simulink model "EdLuTSimulink"  (Simulink 8.1)
settings: Solver=ode3  StartTime=0.0  StopTime=1.  FixedStep=0.002  RelTol=1e-3
undefined symbols (not defined in the file or in its folder): frne
undefined symbols (not defined in the file): context, RRedKuKa, RRedKuKadet
libraries: simulink x1
(part 2 of 2)

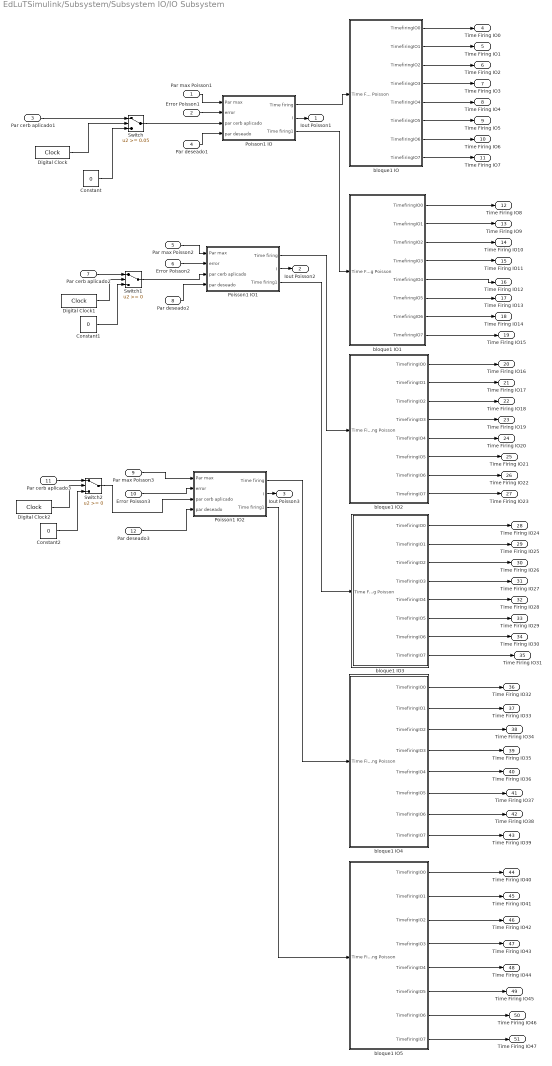
== system EdLuTSimulink/Subsystem/Subsystem IO/IO Subsystem  ==
  Par max Poisson1 : Inport
  Error Poisson1 : Inport  Port=2
  Par cerb aplicado1 : Inport  Port=3
  Par deseado1 : Inport  Port=4
  Par max Poisson2 : Inport  Port=5
  Error Poisson2 : Inport  Port=6
  Par cerb aplicado2 : Inport  Port=7
  Par deseado2 : Inport  Port=8
  Par max Poisson3 : Inport  Port=9
  Error Poisson3 : Inport  Port=10
  Par cerb aplicado3 : Inport  Port=11
  Par deseado3 : Inport  Port=12
  Constant : Constant  Value=0
  Constant1 : Constant  Value=0
  Constant2 : Constant  Value=0
  Digital Clock : DigitalClock  SampleTime=0.002
  Digital Clock1 : DigitalClock  SampleTime=0.002
  Digital Clock2 : DigitalClock  SampleTime=0.002
  Poisson1 IO : Subsystem  mask{a=0.001, b=1, timestep=0.002, firingrate=50}
      mask prompts: a "Valor a del intervalo [a b] para la generación de la poisson"; b "Valor b del intervalo [a b] para la generación de la poisson"; timestep "Tiempo de paso"
  Poisson1 IO1 : Subsystem  mask{a=0.001, b=1, timestep=0.002, firingrate=50}
      mask prompts: a "Valor a del intervalo [a b] para la generación de la poisson"; b "Valor b del intervalo [a b] para la generación de la poisson"; timestep "Tiempo de paso"
  Poisson1 IO2 : Subsystem  mask{a=0.001, b=1, timestep=0.002, firingrate=50}
      mask prompts: a "Valor a del intervalo [a b] para la generación de la poisson"; b "Valor b del intervalo [a b] para la generación de la poisson"; timestep "Tiempo de paso"
  Switch : Switch  Threshold=0.05
  Switch1 : Switch
  Switch2 : Switch
  bloque1 IO : Subsystem
  bloque1 IO1 : Subsystem
  bloque1 IO2 : Subsystem
  bloque1 IO3 : Subsystem
  bloque1 IO4 : Subsystem
  bloque1 IO5 : Subsystem
  Iout Poisson1 : Outport
  Iout Poisson2 : Outport  Port=2
  Iout Poisson3 : Outport  Port=3
  Time Firing IO0 : Outport  Port=4
  Time Firing IO1 : Outport  Port=5
  Time Firing IO2 : Outport  Port=6
  Time Firing IO3 : Outport  Port=7
  Time Firing IO4 : Outport  Port=8
  Time Firing IO5 : Outport  Port=9
  Time Firing IO6 : Outport  Port=10
  Time Firing IO7 : Outport  Port=11
  Time Firing IO8 : Outport  Port=12
  Time Firing IO9 : Outport  Port=13
  Time Firing IO10 : Outport  Port=14
  Time Firing IO11 : Outport  Port=15
  Time Firing IO12 : Outport  Port=16
  Time Firing IO13 : Outport  Port=17
  Time Firing IO14 : Outport  Port=18
  Time Firing IO15 : Outport  Port=19
  Time Firing IO16 : Outport  Port=20
  Time Firing IO17 : Outport  Port=21
  Time Firing IO18 : Outport  Port=22
  Time Firing IO19 : Outport  Port=23
  Time Firing IO20 : Outport  Port=24
  Time Firing IO21 : Outport  Port=25
  Time Firing IO22 : Outport  Port=26
  Time Firing IO23 : Outport  Port=27
  Time Firing IO24 : Outport  Port=28
  Time Firing IO25 : Outport  Port=29
  Time Firing IO26 : Outport  Port=30
  Time Firing IO27 : Outport  Port=31
  Time Firing IO28 : Outport  Port=32
  Time Firing IO29 : Outport  Port=33
  Time Firing IO30 : Outport  Port=34
  Time Firing IO31 : Outport  Port=35
  Time Firing IO32 : Outport  Port=36
  Time Firing IO33 : Outport  Port=37
  Time Firing IO34 : Outport  Port=38
  Time Firing IO35 : Outport  Port=39
  Time Firing IO36 : Outport  Port=40
  Time Firing IO37 : Outport  Port=41
  Time Firing IO38 : Outport  Port=42
  Time Firing IO39 : Outport  Port=43
  Time Firing IO40 : Outport  Port=44
  Time Firing IO41 : Outport  Port=45
  Time Firing IO42 : Outport  Port=46
  Time Firing IO43 : Outport  Port=47
  Time Firing IO44 : Outport  Port=48
  Time Firing IO45 : Outport  Port=49
  Time Firing IO46 : Outport  Port=50
  Time Firing IO47 : Outport  Port=51
  wires:
  Poisson1 IO/1(Time firing) -> bloque1 IO/1(Time Firing Poisson)
  Poisson1 IO/3(Time firing1) -> bloque1 IO1/1(Time Firing Poisson)
  Par max Poisson1/1 -> Poisson1 IO/1(Par max)
  Error Poisson1/1 -> Poisson1 IO/2(error)
  Poisson1 IO/2(I) -> Iout Poisson1/1
  Par deseado1/1 -> Poisson1 IO/4(par deseado)
  Par max Poisson2/1 -> Poisson1 IO1/1(Par max)
  Error Poisson2/1 -> Poisson1 IO1/2(error)
  Par deseado2/1 -> Poisson1 IO1/4(par deseado)
  Poisson1 IO1/3(Time firing1) -> bloque1 IO3/1(Time Firing Poisson)
  bloque1 IO1/1(TimefiringIO0) -> Time Firing IO8/1
  bloque1 IO1/2(TimefiringIO1) -> Time Firing IO9/1
  bloque1 IO1/3(TimefiringIO2) -> Time Firing IO10/1
  bloque1 IO1/4(TimefiringIO3) -> Time Firing IO11/1
  bloque1 IO1/5(TimefiringIO4) -> Time Firing IO12/1
  bloque1 IO1/6(TimefiringIO5) -> Time Firing IO13/1
  bloque1 IO1/7(TimefiringIO6) -> Time Firing IO14/1
  bloque1 IO1/8(TimefiringIO7) -> Time Firing IO15/1
  bloque1 IO2/1(TimefiringIO0) -> Time Firing IO16/1
  bloque1 IO2/2(TimefiringIO1) -> Time Firing IO17/1
  bloque1 IO2/3(TimefiringIO2) -> Time Firing IO18/1
  bloque1 IO2/4(TimefiringIO3) -> Time Firing IO19/1
  bloque1 IO2/5(TimefiringIO4) -> Time Firing IO20/1
  bloque1 IO2/6(TimefiringIO5) -> Time Firing IO21/1
  bloque1 IO2/7(TimefiringIO6) -> Time Firing IO22/1
  bloque1 IO2/8(TimefiringIO7) -> Time Firing IO23/1
  bloque1 IO3/2(TimefiringIO1) -> Time Firing IO25/1
  bloque1 IO3/3(TimefiringIO2) -> Time Firing IO26/1
  bloque1 IO3/4(TimefiringIO3) -> Time Firing IO27/1
  bloque1 IO3/5(TimefiringIO4) -> Time Firing IO28/1
  bloque1 IO3/6(TimefiringIO5) -> Time Firing IO29/1
  bloque1 IO3/7(TimefiringIO6) -> Time Firing IO30/1
  bloque1 IO3/8(TimefiringIO7) -> Time Firing IO31/1
  bloque1 IO3/1(TimefiringIO0) -> Time Firing IO24/1
  Digital Clock/1 -> Switch/2
  Constant/1 -> Switch/3
  Switch/1 -> Poisson1 IO/3(par cerb aplicado)
  Par cerb aplicado2/1 -> Switch1/1
  Digital Clock1/1 -> Switch1/2
  Constant1/1 -> Switch1/3
  Switch1/1 -> Poisson1 IO1/3(par cerb aplicado)
  Par cerb aplicado1/1 -> Switch/1
  Par cerb aplicado3/1 -> Switch2/1
  Digital Clock2/1 -> Switch2/2
  Constant2/1 -> Switch2/3
  Switch2/1 -> Poisson1 IO2/3(par cerb aplicado)
  Par max Poisson3/1 -> Poisson1 IO2/1(Par max)
  Error Poisson3/1 -> Poisson1 IO2/2(error)
  Par deseado3/1 -> Poisson1 IO2/4(par deseado)
  Poisson1 IO2/2(I) -> Iout Poisson3/1
  Poisson1 IO2/1(Time firing) -> bloque1 IO4/1(Time Firing Poisson)
  Poisson1 IO2/3(Time firing1) -> bloque1 IO5/1(Time Firing Poisson)
  bloque1 IO5/1(TimefiringIO0) -> Time Firing IO40/1
  bloque1 IO5/2(TimefiringIO1) -> Time Firing IO41/1
  bloque1 IO5/3(TimefiringIO2) -> Time Firing IO42/1
  bloque1 IO5/4(TimefiringIO3) -> Time Firing IO43/1
  bloque1 IO5/5(TimefiringIO4) -> Time Firing IO44/1
  bloque1 IO5/6(TimefiringIO5) -> Time Firing IO45/1
  bloque1 IO5/7(TimefiringIO6) -> Time Firing IO46/1
  bloque1 IO5/8(TimefiringIO7) -> Time Firing IO47/1
  Poisson1 IO1/2(I) -> Iout Poisson2/1
  Poisson1 IO1/1(Time firing) -> bloque1 IO2/1(Time Firing Poisson)
  bloque1 IO/1(TimefiringIO0) -> Time Firing IO0/1
  bloque1 IO/2(TimefiringIO1) -> Time Firing IO1/1
  bloque1 IO/3(TimefiringIO2) -> Time Firing IO2/1
  bloque1 IO/4(TimefiringIO3) -> Time Firing IO3/1
  bloque1 IO/5(TimefiringIO4) -> Time Firing IO4/1
  bloque1 IO/6(TimefiringIO5) -> Time Firing IO5/1
  bloque1 IO/7(TimefiringIO6) -> Time Firing IO6/1
  bloque1 IO/8(TimefiringIO7) -> Time Firing IO7/1
  bloque1 IO4/1(TimefiringIO0) -> Time Firing IO32/1
  bloque1 IO4/2(TimefiringIO1) -> Time Firing IO33/1
  bloque1 IO4/3(TimefiringIO2) -> Time Firing IO34/1
  bloque1 IO4/4(TimefiringIO3) -> Time Firing IO35/1
  bloque1 IO4/5(TimefiringIO4) -> Time Firing IO36/1
  bloque1 IO4/6(TimefiringIO5) -> Time Firing IO37/1
  bloque1 IO4/7(TimefiringIO6) -> Time Firing IO38/1
  bloque1 IO4/8(TimefiringIO7) -> Time Firing IO39/1

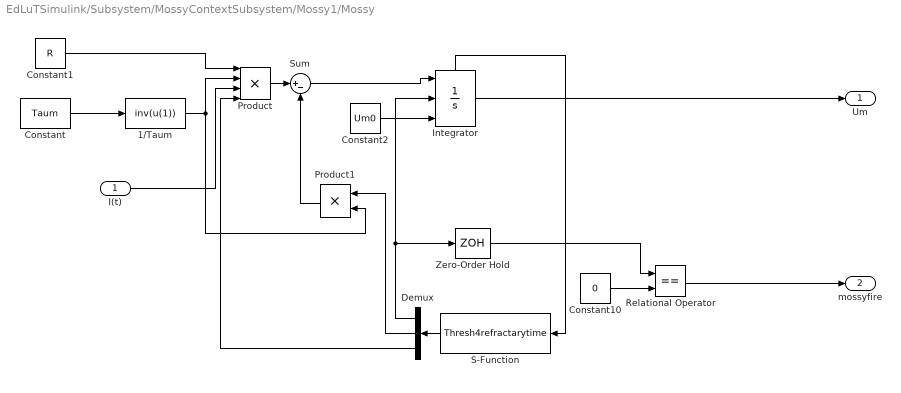
== system EdLuTSimulink/Subsystem/MossyContextSubsystem/Mossy1/Mossy ==
  I(t) : Inport
  1/Taum : MATLABFcn  MATLABFcn=inv(u(1))
  Constant : Constant  Value=Taum
  Constant1 : Constant  Value=R
  Constant10 : Constant  Value=0
  Constant2 : Constant  Value=Um0
  Demux : Demux  Outputs=3
  Integrator : Integrator  ExternalReset=falling  InitialConditionSource=external  LimitOutput=on  UpperSaturationLimit=Uth  LowerSaturationLimit=Ureset  ShowStatePort=on
  Product : Product  Inputs=4  RndMeth=Zero
  Product1 : Product  RndMeth=Zero
  Relational Operator : RelationalOperator  Operator===  OutDataTypeStr=boolean
  S-Function : S-Function  FunctionName=Thresh4refractarytime  Parameters=Uth,Ureset,Trefract  EnableBusSupport=off
  Sum : Sum  Inputs=|+-
  Zero-Order Hold : ZeroOrderHold  SampleTime=0.002
  Um : Outport
  mossyfire : Outport  Port=2
  wires:
  Constant/1 -> 1/Taum/1
  1/Taum/1 -> Product1/2, Product/2
  Constant1/1 -> Product/1
  Product/1 -> Sum/1
  Sum/1 -> Integrator/1
  Integrator/1 -> Um/1
  Product1/1 -> Sum/2
  I(t)/1 -> Product/3
  S-Function/1 -> Demux/1
  Demux/2 -> Product1/1
  Demux/1 -> Integrator/2, Zero-Order Hold/1
  Constant10/1 -> Relational Operator/2
  Relational Operator/1 -> mossyfire/1
  Integrator/State -> S-Function/1
  Constant2/1 -> Integrator/3
  Demux/3 -> Product/4
  Zero-Order Hold/1 -> Relational Operator/1

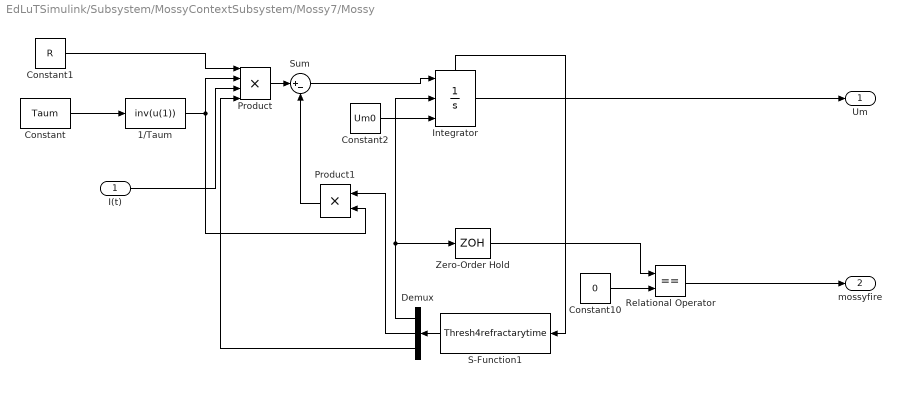
== system EdLuTSimulink/Subsystem/MossyContextSubsystem/Mossy7/Mossy ==
  I(t) : Inport
  1/Taum : MATLABFcn  MATLABFcn=inv(u(1))
  Constant : Constant  Value=Taum
  Constant1 : Constant  Value=R
  Constant10 : Constant  Value=0
  Constant2 : Constant  Value=Um0
  Demux : Demux  Outputs=3
  Integrator : Integrator  ExternalReset=falling  InitialConditionSource=external  LimitOutput=on  UpperSaturationLimit=Uth  LowerSaturationLimit=Ureset  ShowStatePort=on
  Product : Product  Inputs=4  RndMeth=Zero
  Product1 : Product  RndMeth=Zero
  Relational Operator : RelationalOperator  Operator===  OutDataTypeStr=boolean
  S-Function1 : S-Function  FunctionName=Thresh4refractarytime  Parameters=Uth,Ureset,Trefract  EnableBusSupport=off
  Sum : Sum  Inputs=|+-
  Zero-Order Hold : ZeroOrderHold  SampleTime=0.002
  Um : Outport
  mossyfire : Outport  Port=2
  wires:
  Constant/1 -> 1/Taum/1
  1/Taum/1 -> Product1/2, Product/2
  Constant1/1 -> Product/1
  Product/1 -> Sum/1
  Sum/1 -> Integrator/1
  Integrator/1 -> Um/1
  Product1/1 -> Sum/2
  I(t)/1 -> Product/3
  S-Function1/1 -> Demux/1
  Demux/2 -> Product1/1
  Demux/1 -> Integrator/2, Zero-Order Hold/1
  Constant10/1 -> Relational Operator/2
  Relational Operator/1 -> mossyfire/1
  Integrator/State -> S-Function1/1
  Constant2/1 -> Integrator/3
  Demux/3 -> Product/4
  Zero-Order Hold/1 -> Relational Operator/1

== system EdLuTSimulink/Subsystem/MossyInputsSubsystem/Mossy/Mossy ==
  I(t) : Inport
  1/Taum : MATLABFcn  MATLABFcn=inv(u(1))
  Constant : Constant  Value=Taum
  Constant1 : Constant  Value=R
  Constant10 : Constant  Value=0
  Constant2 : Constant  Value=Um0
  Demux : Demux  Outputs=3
  Integrator : Integrator  ExternalReset=falling  InitialConditionSource=external  LimitOutput=on  UpperSaturationLimit=Uth  LowerSaturationLimit=Ureset  ShowStatePort=on
  Product : Product  Inputs=4  RndMeth=Zero
  Product1 : Product  RndMeth=Zero
  Relational Operator : RelationalOperator  Operator===  OutDataTypeStr=boolean
  S-Function : S-Function  FunctionName=ThreshMFsrefractarytime  Parameters=Uth,Ureset,Trefract,NumMFs  EnableBusSupport=off
  Sum : Sum  Inputs=|+-
  Zero-Order Hold : ZeroOrderHold  SampleTime=0.002
  Um : Outport
  mossyfire : Outport  Port=2
  wires:
  Constant/1 -> 1/Taum/1
  1/Taum/1 -> Product1/2, Product/2
  Constant1/1 -> Product/1
  Product/1 -> Sum/1
  Sum/1 -> Integrator/1
  Integrator/1 -> Um/1
  Product1/1 -> Sum/2
  I(t)/1 -> Product/3
  S-Function/1 -> Demux/1
  Demux/2 -> Product1/1
  Demux/1 -> Integrator/2, Zero-Order Hold/1
  Constant10/1 -> Relational Operator/2
  Relational Operator/1 -> mossyfire/1
  Integrator/State -> S-Function/1
  Constant2/1 -> Integrator/3
  Demux/3 -> Product/4
  Zero-Order Hold/1 -> Relational Operator/1

== system EdLuTSimulink/Subsystem/MossyInputsSubsystem/Mossy1/Mossy ==
  I(t) : Inport
  1/Taum : MATLABFcn  MATLABFcn=inv(u(1))
  Constant : Constant  Value=Taum
  Constant1 : Constant  Value=R
  Constant10 : Constant  Value=0
  Constant2 : Constant  Value=Um0
  Demux : Demux  Outputs=3
  Integrator : Integrator  ExternalReset=falling  InitialConditionSource=external  LimitOutput=on  UpperSaturationLimit=Uth  LowerSaturationLimit=Ureset  ShowStatePort=on
  Product : Product  Inputs=4  RndMeth=Zero
  Product1 : Product  RndMeth=Zero
  Relational Operator : RelationalOperator  Operator===  OutDataTypeStr=boolean
  S-Function : S-Function  FunctionName=ThreshMFsrefractarytime  Parameters=Uth,Ureset,Trefract,NumMFs  EnableBusSupport=off
  Sum : Sum  Inputs=|+-
  Zero-Order Hold : ZeroOrderHold  SampleTime=0.002
  Um : Outport
  mossyfire : Outport  Port=2
  wires:
  Constant/1 -> 1/Taum/1
  1/Taum/1 -> Product1/2, Product/2
  Constant1/1 -> Product/1
  Product/1 -> Sum/1
  Sum/1 -> Integrator/1
  Integrator/1 -> Um/1
  Product1/1 -> Sum/2
  I(t)/1 -> Product/3
  S-Function/1 -> Demux/1
  Demux/2 -> Product1/1
  Demux/1 -> Integrator/2, Zero-Order Hold/1
  Constant10/1 -> Relational Operator/2
  Relational Operator/1 -> mossyfire/1
  Integrator/State -> S-Function/1
  Constant2/1 -> Integrator/3
  Demux/3 -> Product/4
  Zero-Order Hold/1 -> Relational Operator/1

== system EdLuTSimulink/Subsystem/MossyInputsSubsystem/Mossy2/Mossy ==
  I(t) : Inport
  1/Taum : MATLABFcn  MATLABFcn=inv(u(1))
  Constant : Constant  Value=Taum
  Constant1 : Constant  Value=R
  Constant10 : Constant  Value=0
  Constant2 : Constant  Value=Um0
  Demux : Demux  Outputs=3
  Integrator : Integrator  ExternalReset=falling  InitialConditionSource=external  LimitOutput=on  UpperSaturationLimit=Uth  LowerSaturationLimit=Ureset  ShowStatePort=on
  Product : Product  Inputs=4  RndMeth=Zero
  Product1 : Product  RndMeth=Zero
  Relational Operator : RelationalOperator  Operator===  OutDataTypeStr=boolean
  S-Function : S-Function  FunctionName=ThreshMFsrefractarytime  Parameters=Uth,Ureset,Trefract,NumMFs  EnableBusSupport=off
  Sum : Sum  Inputs=|+-
  Zero-Order Hold : ZeroOrderHold  SampleTime=0.002
  Um : Outport
  mossyfire : Outport  Port=2
  wires:
  Constant/1 -> 1/Taum/1
  1/Taum/1 -> Product1/2, Product/2
  Constant1/1 -> Product/1
  Product/1 -> Sum/1
  Sum/1 -> Integrator/1
  Integrator/1 -> Um/1
  Product1/1 -> Sum/2
  I(t)/1 -> Product/3
  S-Function/1 -> Demux/1
  Demux/2 -> Product1/1
  Demux/1 -> Integrator/2, Zero-Order Hold/1
  Constant10/1 -> Relational Operator/2
  Relational Operator/1 -> mossyfire/1
  Integrator/State -> S-Function/1
  Constant2/1 -> Integrator/3
  Demux/3 -> Product/4
  Zero-Order Hold/1 -> Relational Operator/1

== system EdLuTSimulink/Subsystem/MossyInputsSubsystem/Mossy3/Mossy ==
  I(t) : Inport
  1/Taum : MATLABFcn  MATLABFcn=inv(u(1))
  Constant : Constant  Value=Taum
  Constant1 : Constant  Value=R
  Constant10 : Constant  Value=0
  Constant2 : Constant  Value=Um0
  Demux : Demux  Outputs=3
  Integrator : Integrator  ExternalReset=falling  InitialConditionSource=external  LimitOutput=on  UpperSaturationLimit=Uth  LowerSaturationLimit=Ureset  ShowStatePort=on
  Product : Product  Inputs=4  RndMeth=Zero
  Product1 : Product  RndMeth=Zero
  Relational Operator : RelationalOperator  Operator===  OutDataTypeStr=boolean
  S-Function : S-Function  FunctionName=ThreshMFsrefractarytime  Parameters=Uth,Ureset,Trefract,NumMFs  EnableBusSupport=off
  Sum : Sum  Inputs=|+-
  Zero-Order Hold : ZeroOrderHold  SampleTime=0.002
  Um : Outport
  mossyfire : Outport  Port=2
  wires:
  Constant/1 -> 1/Taum/1
  1/Taum/1 -> Product1/2, Product/2
  Constant1/1 -> Product/1
  Product/1 -> Sum/1
  Sum/1 -> Integrator/1
  Integrator/1 -> Um/1
  Product1/1 -> Sum/2
  I(t)/1 -> Product/3
  S-Function/1 -> Demux/1
  Demux/2 -> Product1/1
  Demux/1 -> Integrator/2, Zero-Order Hold/1
  Constant10/1 -> Relational Operator/2
  Relational Operator/1 -> mossyfire/1
  Integrator/State -> S-Function/1
  Constant2/1 -> Integrator/3
  Demux/3 -> Product/4
  Zero-Order Hold/1 -> Relational Operator/1

== system EdLuTSimulink/Subsystem/MossyInputsSubsystem/Mossy4/Mossy ==
  I(t) : Inport
  1/Taum : MATLABFcn  MATLABFcn=inv(u(1))
  Constant : Constant  Value=Taum
  Constant1 : Constant  Value=R
  Constant10 : Constant  Value=0
  Constant2 : Constant  Value=Um0
  Demux : Demux  Outputs=3
  Integrator : Integrator  ExternalReset=falling  InitialConditionSource=external  LimitOutput=on  UpperSaturationLimit=Uth  LowerSaturationLimit=Ureset  ShowStatePort=on
  Product : Product  Inputs=4  RndMeth=Zero
  Product1 : Product  RndMeth=Zero
  Relational Operator : RelationalOperator  Operator===  OutDataTypeStr=boolean
  S-Function : S-Function  FunctionName=ThreshMFsrefractarytime  Parameters=Uth,Ureset,Trefract,NumMFs  EnableBusSupport=off
  Sum : Sum  Inputs=|+-
  Zero-Order Hold : ZeroOrderHold  SampleTime=0.002
  Um : Outport
  mossyfire : Outport  Port=2
  wires:
  Constant/1 -> 1/Taum/1
  1/Taum/1 -> Product1/2, Product/2
  Constant1/1 -> Product/1
  Product/1 -> Sum/1
  Sum/1 -> Integrator/1
  Integrator/1 -> Um/1
  Product1/1 -> Sum/2
  I(t)/1 -> Product/3
  S-Function/1 -> Demux/1
  Demux/2 -> Product1/1
  Demux/1 -> Integrator/2, Zero-Order Hold/1
  Constant10/1 -> Relational Operator/2
  Relational Operator/1 -> mossyfire/1
  Integrator/State -> S-Function/1
  Constant2/1 -> Integrator/3
  Demux/3 -> Product/4
  Zero-Order Hold/1 -> Relational Operator/1

== system EdLuTSimulink/Subsystem/MossyInputsSubsystem/Mossy5/Mossy ==
  I(t) : Inport
  1/Taum : MATLABFcn  MATLABFcn=inv(u(1))
  Constant : Constant  Value=Taum
  Constant1 : Constant  Value=R
  Constant10 : Constant  Value=0
  Constant2 : Constant  Value=Um0
  Demux : Demux  Outputs=3
  Integrator : Integrator  ExternalReset=falling  InitialConditionSource=external  LimitOutput=on  UpperSaturationLimit=Uth  LowerSaturationLimit=Ureset  ShowStatePort=on
  Product : Product  Inputs=4  RndMeth=Zero
  Product1 : Product  RndMeth=Zero
  Relational Operator : RelationalOperator  Operator===  OutDataTypeStr=boolean
  S-Function : S-Function  FunctionName=ThreshMFsrefractarytime  Parameters=Uth,Ureset,Trefract,NumMFs  EnableBusSupport=off
  Sum : Sum  Inputs=|+-
  Zero-Order Hold : ZeroOrderHold  SampleTime=0.002
  Um : Outport
  mossyfire : Outport  Port=2
  wires:
  Constant/1 -> 1/Taum/1
  1/Taum/1 -> Product1/2, Product/2
  Constant1/1 -> Product/1
  Product/1 -> Sum/1
  Sum/1 -> Integrator/1
  Integrator/1 -> Um/1
  Product1/1 -> Sum/2
  I(t)/1 -> Product/3
  S-Function/1 -> Demux/1
  Demux/2 -> Product1/1
  Demux/1 -> Integrator/2, Zero-Order Hold/1
  Constant10/1 -> Relational Operator/2
  Relational Operator/1 -> mossyfire/1
  Integrator/State -> S-Function/1
  Constant2/1 -> Integrator/3
  Demux/3 -> Product/4
  Zero-Order Hold/1 -> Relational Operator/1

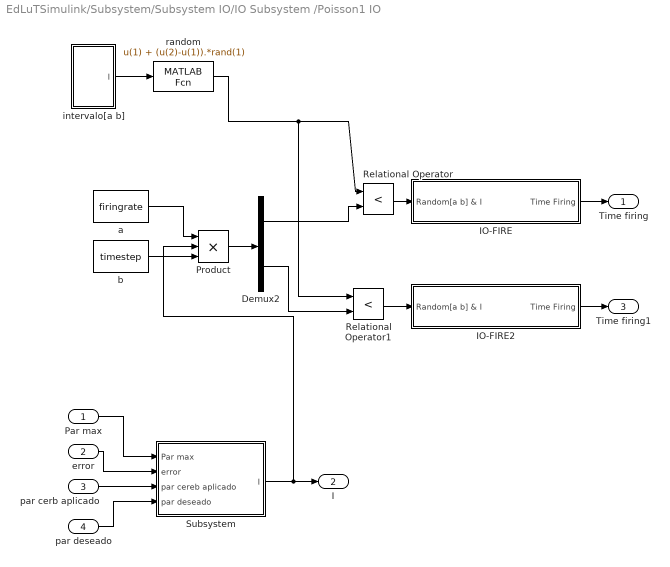
== system EdLuTSimulink/Subsystem/Subsystem IO/IO Subsystem /Poisson1 IO ==
  Par max : Inport
  error : Inport  Port=2
  par cerb aplicado : Inport  Port=3
  par deseado : Inport  Port=4
  Demux2 : Demux  Outputs=2
  IO-FIRE : Subsystem
  IO-FIRE2 : Subsystem
  Product : Product  Inputs=3  RndMeth=Zero
  Relational Operator : RelationalOperator  Operator=<  OutDataTypeStr=boolean
  Relational Operator1 : RelationalOperator  Operator=<  OutDataTypeStr=boolean
  Subsystem : Subsystem
  a : Constant  Value=firingrate
  b : Constant  Value=timestep
  intervalo[a b] : Subsystem
  random : MATLABFcn  MATLABFcn=u(1) + (u(2)-u(1)).*rand(1)
  Time firing : Outport
  I : Outport  Port=2
  Time firing1 : Outport  Port=3
  wires:
  intervalo[a b]/1(I) -> random/1
  par cerb aplicado/1 -> Subsystem/3(par cereb aplicado)
  Par max/1 -> Subsystem/1(Par max)
  error/1 -> Subsystem/2(error)
  par deseado/1 -> Subsystem/4(par deseado)
  Subsystem/1(I) -> I/1, Product/2
  Demux2/1 -> Relational Operator/2
  Demux2/2 -> Relational Operator1/2
  a/1 -> Product/1
  Relational Operator/1 -> IO-FIRE/1(Random[a b] & I)
  IO-FIRE/1(Time Firing) -> Time firing/1
  Relational Operator1/1 -> IO-FIRE2/1(Random[a b] & I)
  Product/1 -> Demux2/1
  b/1 -> Product/3
  random/1 -> Relational Operator/1, Relational Operator1/1
  IO-FIRE2/1(Time Firing) -> Time firing1/1

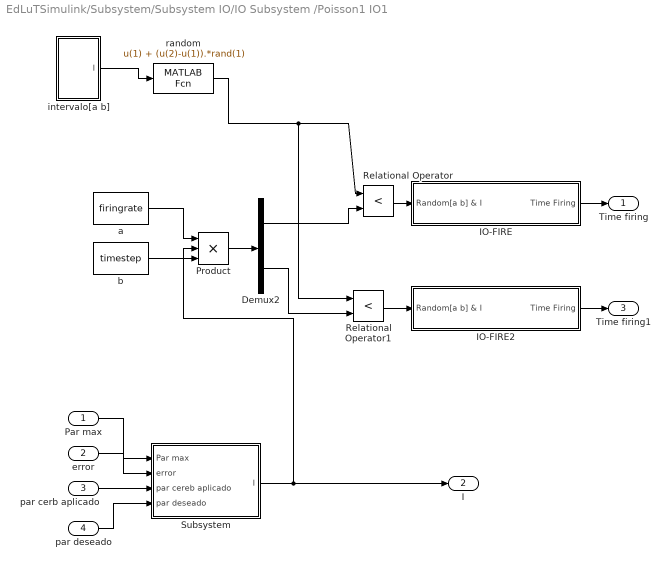
== system EdLuTSimulink/Subsystem/Subsystem IO/IO Subsystem /Poisson1 IO1 ==
  Par max : Inport
  error : Inport  Port=2
  par cerb aplicado : Inport  Port=3
  par deseado : Inport  Port=4
  Demux2 : Demux  Outputs=2
  IO-FIRE : Subsystem
  IO-FIRE2 : Subsystem
  Product : Product  Inputs=3  RndMeth=Zero
  Relational Operator : RelationalOperator  Operator=<  OutDataTypeStr=boolean
  Relational Operator1 : RelationalOperator  Operator=<  OutDataTypeStr=boolean
  Subsystem : Subsystem
  a : Constant  Value=firingrate
  b : Constant  Value=timestep
  intervalo[a b] : Subsystem
  random : MATLABFcn  MATLABFcn=u(1) + (u(2)-u(1)).*rand(1)
  Time firing : Outport
  I : Outport  Port=2
  Time firing1 : Outport  Port=3
  wires:
  intervalo[a b]/1(I) -> random/1
  Par max/1 -> Subsystem/1(Par max)
  par deseado/1 -> Subsystem/4(par deseado)
  Subsystem/1(I) -> I/1, Product/2
  Demux2/1 -> Relational Operator/2
  Demux2/2 -> Relational Operator1/2
  a/1 -> Product/1
  Relational Operator/1 -> IO-FIRE/1(Random[a b] & I)
  IO-FIRE/1(Time Firing) -> Time firing/1
  Relational Operator1/1 -> IO-FIRE2/1(Random[a b] & I)
  Product/1 -> Demux2/1
  b/1 -> Product/3
  random/1 -> Relational Operator/1, Relational Operator1/1
  IO-FIRE2/1(Time Firing) -> Time firing1/1
  par cerb aplicado/1 -> Subsystem/3(par cereb aplicado)
  error/1 -> Subsystem/2(error)

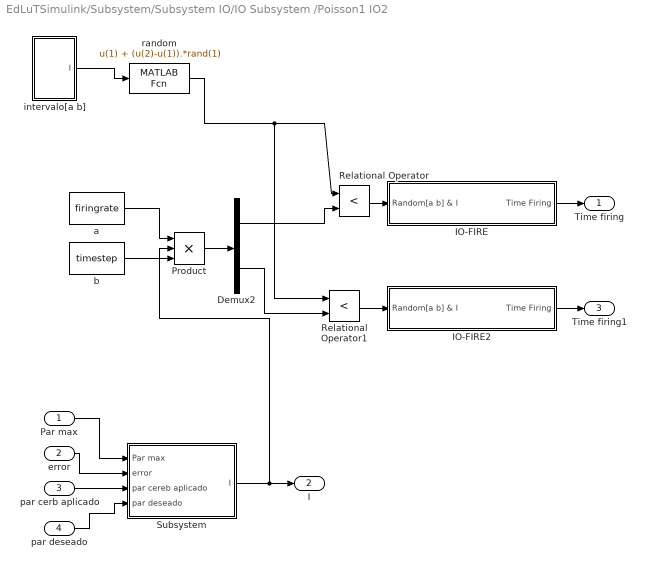
== system EdLuTSimulink/Subsystem/Subsystem IO/IO Subsystem /Poisson1 IO2 ==
  Par max : Inport
  error : Inport  Port=2
  par cerb aplicado : Inport  Port=3
  par deseado : Inport  Port=4
  Demux2 : Demux  Outputs=2
  IO-FIRE : Subsystem
  IO-FIRE2 : Subsystem
  Product : Product  Inputs=3  RndMeth=Zero
  Relational Operator : RelationalOperator  Operator=<  OutDataTypeStr=boolean
  Relational Operator1 : RelationalOperator  Operator=<  OutDataTypeStr=boolean
  Subsystem : Subsystem
  a : Constant  Value=firingrate
  b : Constant  Value=timestep
  intervalo[a b] : Subsystem
  random : MATLABFcn  MATLABFcn=u(1) + (u(2)-u(1)).*rand(1)
  Time firing : Outport
  I : Outport  Port=2
  Time firing1 : Outport  Port=3
  wires:
  intervalo[a b]/1(I) -> random/1
  Par max/1 -> Subsystem/1(Par max)
  error/1 -> Subsystem/2(error)
  par deseado/1 -> Subsystem/4(par deseado)
  Subsystem/1(I) -> I/1, Product/2
  Demux2/1 -> Relational Operator/2
  Demux2/2 -> Relational Operator1/2
  a/1 -> Product/1
  Relational Operator/1 -> IO-FIRE/1(Random[a b] & I)
  IO-FIRE/1(Time Firing) -> Time firing/1
  Relational Operator1/1 -> IO-FIRE2/1(Random[a b] & I)
  Product/1 -> Demux2/1
  b/1 -> Product/3
  random/1 -> Relational Operator/1, Relational Operator1/1
  IO-FIRE2/1(Time Firing) -> Time firing1/1
  par cerb aplicado/1 -> Subsystem/3(par cereb aplicado)

== system EdLuTSimulink/Subsystem/Subsystem IO/IO Subsystem /bloque1 IO ==
  Time Firing Poisson : Inport
  TimefiringIO0 : Outport
  TimefiringIO1 : Outport  Port=2
  TimefiringIO2 : Outport  Port=3
  TimefiringIO3 : Outport  Port=4
  TimefiringIO4 : Outport  Port=5
  TimefiringIO5 : Outport  Port=6
  TimefiringIO6 : Outport  Port=7
  TimefiringIO7 : Outport  Port=8
  wires:
  Time Firing Poisson/1 -> TimefiringIO0/1, TimefiringIO1/1, TimefiringIO2/1, TimefiringIO3/1, TimefiringIO4/1, TimefiringIO5/1, TimefiringIO6/1, TimefiringIO7/1

== system EdLuTSimulink/Subsystem/Subsystem IO/IO Subsystem /bloque1 IO1 ==
  Time Firing Poisson : Inport
  TimefiringIO0 : Outport
  TimefiringIO1 : Outport  Port=2
  TimefiringIO2 : Outport  Port=3
  TimefiringIO3 : Outport  Port=4
  TimefiringIO4 : Outport  Port=5
  TimefiringIO5 : Outport  Port=6
  TimefiringIO6 : Outport  Port=7
  TimefiringIO7 : Outport  Port=8
  wires:
  Time Firing Poisson/1 -> TimefiringIO2/1, TimefiringIO0/1, TimefiringIO1/1, TimefiringIO3/1, TimefiringIO4/1, TimefiringIO5/1, TimefiringIO7/1, TimefiringIO6/1

== system EdLuTSimulink/Subsystem/Subsystem IO/IO Subsystem /bloque1 IO2 ==
  Time Firing Poisson : Inport
  TimefiringIO0 : Outport
  TimefiringIO1 : Outport  Port=2
  TimefiringIO2 : Outport  Port=3
  TimefiringIO3 : Outport  Port=4
  TimefiringIO4 : Outport  Port=5
  TimefiringIO5 : Outport  Port=6
  TimefiringIO6 : Outport  Port=7
  TimefiringIO7 : Outport  Port=8
  wires:
  Time Firing Poisson/1 -> TimefiringIO0/1, TimefiringIO1/1, TimefiringIO2/1, TimefiringIO3/1, TimefiringIO4/1, TimefiringIO5/1, TimefiringIO6/1, TimefiringIO7/1

== system EdLuTSimulink/Subsystem/Subsystem IO/IO Subsystem /bloque1 IO3 ==
  Time Firing Poisson : Inport
  TimefiringIO0 : Outport
  TimefiringIO1 : Outport  Port=2
  TimefiringIO2 : Outport  Port=3
  TimefiringIO3 : Outport  Port=4
  TimefiringIO4 : Outport  Port=5
  TimefiringIO5 : Outport  Port=6
  TimefiringIO6 : Outport  Port=7
  TimefiringIO7 : Outport  Port=8
  wires:
  Time Firing Poisson/1 -> TimefiringIO0/1, TimefiringIO1/1, TimefiringIO2/1, TimefiringIO3/1, TimefiringIO4/1, TimefiringIO5/1, TimefiringIO6/1, TimefiringIO7/1

== system EdLuTSimulink/Subsystem/Subsystem IO/IO Subsystem /bloque1 IO4 ==
  Time Firing Poisson : Inport
  TimefiringIO0 : Outport
  TimefiringIO1 : Outport  Port=2
  TimefiringIO2 : Outport  Port=3
  TimefiringIO3 : Outport  Port=4
  TimefiringIO4 : Outport  Port=5
  TimefiringIO5 : Outport  Port=6
  TimefiringIO6 : Outport  Port=7
  TimefiringIO7 : Outport  Port=8
  wires:
  Time Firing Poisson/1 -> TimefiringIO0/1, TimefiringIO1/1, TimefiringIO2/1, TimefiringIO3/1, TimefiringIO4/1, TimefiringIO5/1, TimefiringIO6/1, TimefiringIO7/1

== system EdLuTSimulink/Subsystem/Subsystem IO/IO Subsystem /bloque1 IO5 ==
  Time Firing Poisson : Inport
  TimefiringIO0 : Outport
  TimefiringIO1 : Outport  Port=2
  TimefiringIO2 : Outport  Port=3
  TimefiringIO3 : Outport  Port=4
  TimefiringIO4 : Outport  Port=5
  TimefiringIO5 : Outport  Port=6
  TimefiringIO6 : Outport  Port=7
  TimefiringIO7 : Outport  Port=8
  wires:
  Time Firing Poisson/1 -> TimefiringIO0/1, TimefiringIO1/1, TimefiringIO2/1, TimefiringIO3/1, TimefiringIO4/1, TimefiringIO5/1, TimefiringIO6/1, TimefiringIO7/1

== system EdLuTSimulink/Subsystem/Subsystem IO/IO Subsystem /Poisson1 IO/IO-FIRE ==
  Random[a b] & I : Inport
  Constant : Constant  OutDataTypeStr=boolean
  Constant1 : Constant  Value=0  OutDataTypeStr=boolean
  Switch3 : Switch  Criteria=u2 > Threshold
  Time Firing : Outport
  wires:
  Switch3/1 -> Time Firing/1
  Random[a b] & I/1 -> Switch3/2
  Constant1/1 -> Switch3/3
  Constant/1 -> Switch3/1

== system EdLuTSimulink/Subsystem/Subsystem IO/IO Subsystem /Poisson1 IO/IO-FIRE2 ==
  Random[a b] & I : Inport
  Constant : Constant  OutDataTypeStr=boolean
  Constant1 : Constant  Value=0  OutDataTypeStr=boolean
  Switch3 : Switch  Criteria=u2 > Threshold
  Time Firing : Outport
  wires:
  Switch3/1 -> Time Firing/1
  Random[a b] & I/1 -> Switch3/2
  Constant1/1 -> Switch3/3
  Constant/1 -> Switch3/1

== system EdLuTSimulink/Subsystem/Subsystem IO/IO Subsystem /Poisson1 IO/Subsystem ==
  Par max : Inport
  error : Inport  Port=2
  par cereb aplicado : Inport  Port=3
  par deseado : Inport  Port=4
  Mux2 : Mux
  S-Function : S-Function  FunctionName=errormanagementmod  EnableBusSupport=off
  I : Outport
  wires:
  Par max/1 -> Mux2/1
  error/1 -> Mux2/2
  par cereb aplicado/1 -> Mux2/3
  S-Function/1 -> I/1
  par deseado/1 -> Mux2/4
  Mux2/1 -> S-Function/1

== system EdLuTSimulink/Subsystem/Subsystem IO/IO Subsystem /Poisson1 IO/intervalo[a b] ==
  Mux5 : Mux  Inputs=2
  a : Constant  Value=a
  b : Constant  Value=b
  I : Outport
  wires:
  a/1 -> Mux5/1
  b/1 -> Mux5/2
  Mux5/1 -> I/1

== system EdLuTSimulink/Subsystem/Subsystem IO/IO Subsystem /Poisson1 IO1/IO-FIRE ==
  Random[a b] & I : Inport
  Constant : Constant  OutDataTypeStr=boolean
  Constant1 : Constant  Value=0  OutDataTypeStr=boolean
  Switch3 : Switch  Criteria=u2 > Threshold
  Time Firing : Outport
  wires:
  Switch3/1 -> Time Firing/1
  Random[a b] & I/1 -> Switch3/2
  Constant1/1 -> Switch3/3
  Constant/1 -> Switch3/1

== system EdLuTSimulink/Subsystem/Subsystem IO/IO Subsystem /Poisson1 IO1/IO-FIRE2 ==
  Random[a b] & I : Inport
  Constant : Constant  OutDataTypeStr=boolean
  Constant1 : Constant  Value=0  OutDataTypeStr=boolean
  Switch3 : Switch  Criteria=u2 > Threshold
  Time Firing : Outport
  wires:
  Switch3/1 -> Time Firing/1
  Random[a b] & I/1 -> Switch3/2
  Constant1/1 -> Switch3/3
  Constant/1 -> Switch3/1

== system EdLuTSimulink/Subsystem/Subsystem IO/IO Subsystem /Poisson1 IO1/Subsystem ==
  Par max : Inport
  error : Inport  Port=2
  par cereb aplicado : Inport  Port=3
  par deseado : Inport  Port=4
  Mux2 : Mux
  S-Function : S-Function  FunctionName=errormanagementmod  EnableBusSupport=off
  I : Outport
  wires:
  Par max/1 -> Mux2/1
  error/1 -> Mux2/2
  par cereb aplicado/1 -> Mux2/3
  S-Function/1 -> I/1
  par deseado/1 -> Mux2/4
  Mux2/1 -> S-Function/1

== system EdLuTSimulink/Subsystem/Subsystem IO/IO Subsystem /Poisson1 IO1/intervalo[a b] ==
  Mux5 : Mux  Inputs=2
  a : Constant  Value=a
  b : Constant  Value=b
  I : Outport
  wires:
  a/1 -> Mux5/1
  b/1 -> Mux5/2
  Mux5/1 -> I/1

== system EdLuTSimulink/Subsystem/Subsystem IO/IO Subsystem /Poisson1 IO2/IO-FIRE ==
  Random[a b] & I : Inport
  Constant : Constant  OutDataTypeStr=boolean
  Constant1 : Constant  Value=0  OutDataTypeStr=boolean
  Switch3 : Switch  Criteria=u2 > Threshold
  Time Firing : Outport
  wires:
  Switch3/1 -> Time Firing/1
  Random[a b] & I/1 -> Switch3/2
  Constant1/1 -> Switch3/3
  Constant/1 -> Switch3/1

== system EdLuTSimulink/Subsystem/Subsystem IO/IO Subsystem /Poisson1 IO2/IO-FIRE2 ==
  Random[a b] & I : Inport
  Constant : Constant  OutDataTypeStr=boolean
  Constant1 : Constant  Value=0  OutDataTypeStr=boolean
  Switch3 : Switch  Criteria=u2 > Threshold
  Time Firing : Outport
  wires:
  Switch3/1 -> Time Firing/1
  Random[a b] & I/1 -> Switch3/2
  Constant1/1 -> Switch3/3
  Constant/1 -> Switch3/1

== system EdLuTSimulink/Subsystem/Subsystem IO/IO Subsystem /Poisson1 IO2/Subsystem ==
  Par max : Inport
  error : Inport  Port=2
  par cereb aplicado : Inport  Port=3
  par deseado : Inport  Port=4
  Mux2 : Mux
  S-Function : S-Function  FunctionName=errormanagementmod  EnableBusSupport=off
  I : Outport
  wires:
  Par max/1 -> Mux2/1
  error/1 -> Mux2/2
  par cereb aplicado/1 -> Mux2/3
  S-Function/1 -> I/1
  par deseado/1 -> Mux2/4
  Mux2/1 -> S-Function/1

== system EdLuTSimulink/Subsystem/Subsystem IO/IO Subsystem /Poisson1 IO2/intervalo[a b] ==
  Mux5 : Mux  Inputs=2
  a : Constant  Value=a
  b : Constant  Value=b
  I : Outport
  wires:
  a/1 -> Mux5/1
  b/1 -> Mux5/2
  Mux5/1 -> I/1
